simulink model "quad_linearized_ss"  (R2015b)
settings: Solver=VariableStepAuto  StartTime=0.0  StopTime=20  RelTol=1e-3
settings Model: Creator=zachn  LastModifiedBy=zachn

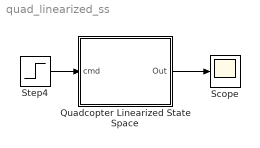
== system quad_linearized_ss ==
  Quadcopter Linearized State Space : Subsystem  mask{m=0.5, i_xyz=[5e-3, 5e-3, 5e-3], g=9.88, A=0, B=0, C=0, D=0}
      mask prompts: m "Mass"; i_xyz "Moment of Inertia Ixyz"; g "Gravity (mm/s^2)"; A "A Matrix"; B "B Matrix"; C "C Matrix"; D "D Matrix"
      mask init:
      | A = [   zeros(3,3), eye(3,3), zeros(3,6)    ; ...
      |         zeros(3,12)                         ; ...
      |         0, -g, zeros(1,10)                  ; ...
      |         g, zeros(1,11)                      ; ...
      |         zeros(1,12)                         ; ...
      |         zeros(3,6), eye(3,3), zeros(3,3)      ...
      |     ];
      | 
      | B = [   zeros(3,4)              ; ...
      |         0, 1/i_xyz(1), 0, 0     ; ...
      |         0, 0, 1/i_xyz(2), 0     ; ...
      |         0, 0, 0, 1/i_xyz(3)     ; ...
      |         zeros(2,4)              ; ...
      |         1/m, 0, 0, 0            ; ...
      |         zeros(3,4)                ...
      |     ];
      | 
      | C = [   zeros(1,9), 1, 0, 0     ; ...
      |         zeros(1,10), 1, 0       ; ...
      |         zeros(1,11), 1          ; ...
      |         0, 0, 1, zeros(1,9)       ...
      |      ];
      |  
      |  D = [  zeros(4,4) ];
      mask DialogControl DescGroupVar Prompt: QUADCOPTA
      mask DialogControl DescTextVar Prompt: Linearized state space model of a four rotor quadcopter.
      mask DialogControl Control2 Prompt: GET TO THE QUADCOPTA!!!
      mask DialogControl Control2 Callback: web www.youtube.com/watch?v=Xs_OacEq2Sk
      mask DialogControl Container4 Prompt: System Parameters
  Scope : Scope
  Step4 : Step  Time=[1;2;3;4]  Before=[0;0;0;0]  After=[1;1;1;1]  SampleTime=0  VectorParams1D=off
  wires:
  Step4/1 -> Quadcopter Linearized State Space/1(cmd)
  Quadcopter Linearized State Space/1(Out) -> Scope/1

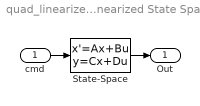
== system quad_linearized_ss/Quadcopter Linearized State Space ==
  cmd : Inport
  State-Space : StateSpace  A=A  B=B  C=C  D=D  X0=0
  Out : Outport
  wires:
  cmd/1 -> State-Space/1
  State-Space/1 -> Out/1
